simulink model "Bicycle_model_nonlinear_constrained"  (R2020b)
settings: Solver=ode15s  StartTime=0.0  StopTime=10.0  RelTol=1e-3
InitFcn:
  | mdl = 'Bicycle_model_nonlinear_constrained';
  | 
  | wks = get_param(mdl, 'ModelWorkspace');
  | 
  | vals_struct_front = load('lateral_data_lut_FRONT.mat');
  | sa_x_front = vals_struct_front.sa_x;
  | load_y_front = vals_struct_front.load_y;
  | %sa_x_front = sa_x_front'*ones(1, length(load_y_front));
  | load_y_front = flip(load_y_front);
  | %load_y_front = ones(size(sa_x_front, 1), 1)*load_y_front;
  | lateral_coeff_front = vals_struct_front.lat_coeff;
  | lateral_coeff_front = fliplr(lateral_coeff_front);
  | aligning_torque_front = vals_struct_front.aligning_torque;
  | aligning_torque_front = fliplr(aligning_torque_front);
  | assignin(wks, 'sa_x_front', sa_x_front);
  | assignin(wks, 'load_y_front', load_y_front);
  | assignin(wks, 'lateral_coeff_front', lateral_coeff_front);
  | assignin(wks, 'aligning_torque_front', aligning_torque_front);
  | 
  | vals_struct_rear = load('lateral_data_lut_REAR.mat');
  | sa_x_rear = vals_struct_rear.sa_x;
  | load_y_rear = vals_struct_rear.load_y;
  | %sa_x_rear = sa_x_rear'*ones(1, length(load_y_rear));
  | load_y_rear = flip(load_y_rear);
  | %load_y_rear = ones(size(sa_x_rear, 1), 1)*load_y_rear;
  | lateral_coeff_rear = vals_struct_rear.lat_coeff;
  | lateral_coeff_rear = fliplr(lateral_coeff_rear);
  | aligning_torque_rear = vals_struct_rear.aligning_torque;
  | aligning_torque_rear = fliplr(aligning_torque_rear);
  | assignin(wks, 'sa_x_rear', sa_x_rear);
  | assignin(wks, 'load_y_rear', load_y_rear);
  | assignin(wks, 'lateral_coeff_rear', lateral_coeff_rear);
  | assignin(wks, 'aligning_torque_rear', aligning_torque_rear);
model workspace (MAT data in the model file):
  Gravity : Simulink.Parameter (value not decoded)
  Mass : Simulink.Parameter (value not decoded)
  Weight_dist : Simulink.Parameter (value not decoded)
  Wheelbase : Simulink.Parameter (value not decoded)
  aligning_torque_front = [-41.5540960755 -41.5662624888 -41.5807188002 -41.5975229416 -41.6167266751 -41.6383748526 -41.6625046744 -41.6891449542 -41.7183154014 -41.7500259272 -41.7842759867 -41.8210539664 ... (18361 elements, 301x61)]
  aligning_torque_rear = [-18.1434786147 -17.5139711055 -16.8077956028 -16.0208528857 -15.1497738315 -14.1923038543 -13.1478032051 -12.0178890979 -10.8072479379 -9.52464615821 -8.18416446104 -6.80666977097 ... (18361 elements, 301x61)]
  lateral_coeff_front = [-2.08355014577 -2.08846565202 -2.09327995784 -2.09799213228 -2.10260121652 -2.10710622309 -2.11150613503 -2.11579990501 -2.11998645448 -2.1240646727 -2.12803341584 -2.13189150601 ... (18361 elements, 301x61)]
  lateral_coeff_rear = [-2.53828292724 -2.53442829982 -2.53054773666 -2.5266407201 -2.52270671872 -2.51874518685 -2.51475556411 -2.51073727486 -2.50668972773 -2.50261231503 -2.49850441218 -2.49436537715 ... (18361 elements, 301x61)]
  load_y_front = [-1200 -1180 -1160 -1140 -1120 -1100 -1080 -1060 -1040 -1020 -1000 -980 ... (61 elements, 1x61)]
  load_y_rear = [-1200 -1180 -1160 -1140 -1120 -1100 -1080 -1060 -1040 -1020 -1000 -980 ... (61 elements, 1x61)]
  sa_x_front = [-0.261799387799 -0.260054058547 -0.258308729295 -0.256563400043 -0.254818070791 -0.253072741539 -0.251327412287 -0.249582083035 -0.247836753783 -0.246091424531 -0.244346095279 -0.242600766027 ... (301 elements, 1x301)]
  sa_x_rear = [-0.261799387799 -0.260054058547 -0.258308729295 -0.256563400043 -0.254818070791 -0.253072741539 -0.251327412287 -0.249582083035 -0.247836753783 -0.246091424531 -0.244346095279 -0.242600766027 ... (301 elements, 1x301)]
symbols that are objects in the model workspace (value not decoded): Gravity, Mass, Weight_dist, Wheelbase
libraries: simulink_extras x4
(part 2 of 2)

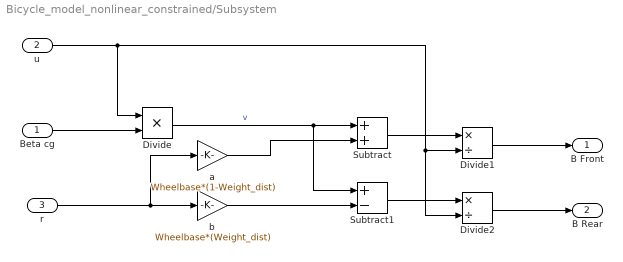
== system Bicycle_model_nonlinear_constrained/Subsystem ==
  Beta cg : Inport
  u : Inport  Port=2
  r : Inport  Port=3
  Divide : Product  Inputs=**
  Divide1 : Product  Inputs=*/
  Divide2 : Product  Inputs=*/
  Subtract : Sum
  Subtract1 : Sum  Inputs=+-
  a : Gain  Gain=Wheelbase*(1-Weight_dist)
  b : Gain  Gain=Wheelbase*(Weight_dist)
  B Front : Outport
  B Rear : Outport  Port=2
  wires:
  Divide/1 -> Subtract1/1, Subtract/1  "v"
  u/1 -> Divide/1, Divide2/2, Divide1/2
  r/1 -> a/1, b/1
  a/1 -> Subtract/2
  b/1 -> Subtract1/2
  Subtract/1 -> Divide1/1
  Subtract1/1 -> Divide2/1
  Divide1/1 -> B Front/1
  Divide2/1 -> B Rear/1
  Beta cg/1 -> Divide/2
